simulink model "KD_cl_harness_cl_ouports_added"  (R2015b)
settings: Solver=ode45  StartTime=0  StopTime=inf  FixedStep=0.01  MaxStep=0.005  RelTol=1e-5  AbsTol=1e-5
undefined symbols (not defined in the file or in its folder): A2, bin_vec, c_0, c_1000, c_1000inv, c_100inv, c_1d2p4, c_1p7, c_4400inv, c_5500inv, c_80, c_compmap, c_ctok, c_fflow_max, c_fflow_min, c_filt, c_flowdiv, c_flowmin, c_flowmult, c_inf, c_km1d2k, c_n1, c_p00001, c_p01, c_p1e9, c_p4d1p4, c_pincomp, c_rair, c_roacorr, c_rpmtoradpers, c_svrthrottle1, c_svrthrottle2, c_svrthrottlearg, c_svrthrottlebeta, c_vnliftmax, c_vnliftmin, cl_offset, clff, Coefs, const, const_exhat, const_vec, Dual_array, dual_zero, egr_ecu_ff, expcon, f_mat, gs_jul, HQP_eps, HQP_INF, HQP_saturation, IV, L2, length_L, maxL, mHQP_saturation, minL, Newton, nRed, num_constraints ... (+22)
libraries: simulink x33
(part 6 of 6)

== system KD_cl_harness_cl_ouports_added/ctrl_rb_explicit_20140220_v6_simp/ntremap/remap_wt_to_map/ThrottleModel1/AirModel_map_use/Forward_Flow/For_Iterator_Subsystem ==
  u : Inport
  sv1 : Inport  Port=2
  sv2 : Inport  Port=3
  arg : Inport  Port=4
  beta : Inport  Port=5
  Demux : Demux  Outputs=2
  Divide : Product  Inputs=*/
  For Iterator : ForIterator  ResetStates=reset  IterationLimit=SVR_EGR_exhat.num_SV
  Gain : Gain  Gain=100
      settings: AttributesFormatString=%<Gain>
  Product{,1..3} (4 alike) : Product  RndMeth=Zero
  Saturation1 : Saturate  UpperLimit=9  LowerLimit=1
      settings: AttributesFormatString=%<LowerLimit>\n%<UpperLimit>
  Selector : Selector  InputPortWidth=SVR_EGR_exhat.num_SV  IndexOptions=Index vector (port)  Indices=[1 3]  OutputSizes=1
  Selector1 : Selector  InputPortWidth=SVR_EGR_exhat.num_SV  IndexOptions=Index vector (port)  Indices=[1 3]  OutputSizes=1
  Selector2 : Selector  InputPortWidth=SVR_EGR_exhat.num_SV  IndexOptions=Index vector (port)  Indices=[1 3]  OutputSizes=1
  Sum : Sum  Inputs=|-+
  Sum1 : Sum  Inputs=+-|
  Sum2 : Sum  Inputs=-|-
  Sum3 : Sum  Inputs=++|
  Unit Delay : UnitDelay  SampleTime=-1
  exp Lookup Table : Lookup  InputValues=SVR_EGR_exhat.exp.x  Table=SVR_EGR_exhat.exp.y  LookUpMeth=Interpolation-Use End Values
      settings: AttributesFormatString=%<LookUpMeth>\n%<InputValues>
  ba : Outport  OutDataTypeStr=single
  sat_out-65 : Outport  Port=2
  wires:
  exp Lookup Table/1 -> Product3/1
  Divide/1 -> exp Lookup Table/1
  Unit Delay/1 -> Sum3/1
  sv1/1 -> Selector/1
  sv2/1 -> Selector1/1
  beta/1 -> Selector2/1
  u/1 -> Demux/1
  Selector/1 -> Sum/1
  Demux/1 -> Sum/2
  Selector1/1 -> Sum1/2
  Demux/2 -> Sum1/1
  Sum/1 -> Product/1, Product/2
  Sum1/1 -> Product1/1, Product1/2
  Product/1 -> Sum2/1
  Product1/1 -> Sum2/2
  Sum2/1 -> Divide/1
  arg/1 -> Product2/1, Product2/2
  Product2/1 -> Gain/1
  Gain/1 -> Divide/2
  Selector2/1 -> Product3/2
  Product3/1 -> Sum3/2
  Sum3/1 -> Unit Delay/1, ba/1
  [iter] -> Selector/2
  [iter] -> Selector1/2
  [iter] -> Selector2/2
  For Iterator/1 -> Saturation1/1, sat_out-65/1
  Saturation1/1 -> [iter]

== matlab function KD_cl_harness_cl_ouports_added/EGR Valve/SVR EGR/EGR_model/Air Model_map_use/Forward-Flow/SVR_EGR ==
  data: u input; B_A_spd output; num_SV input; Beta input; SV input; arg input
function B_A_spd = fcn(u, num_SV, Beta, SV, arg)
%#eml
Kern=zeros(length(SV),1);
    for n=1:num_SV
        v = SV(n,:).';
        Kern(n)=exp(-(u-v)'*(u-v)/(50*(2*arg^2)));
    end
B_A_spd = Beta.'*Kern;

== matlab function KD_cl_harness_cl_ouports_added/Turbine/TurbineMap/TurbineMAP1 ==
  data: turb_pres_ratio input; omega_turbo input; p_in_turb input; T_ambient input; T_exh_man input; VNlift input; W_turbine_sim output; Turb_Constants input; TurbFlowCoefs input; TurbTempCoefs input; T_out_turbine output; eta_turb output; A_turbine output; phi output; delta_T_Turbo output; Tq_turbine output
 function [W_turbine_sim, T_out_turbine,eta_turb,A_turbine,phi,delta_T_Turbo,Tq_turbine] = TurbineMap(turb_pres_ratio,omega_turbo,p_in_turb,T_ambient,T_exh_man,VNlift,Turb_Constants, TurbFlowCoefs, TurbTempCoefs)

%% Reference: Turbocharger modelling for Automotive Control Applications by Paul Moraal and Ilya Kolmanovsky
% if T_exh_man <= 0
%     a = 1;
% end
Dia_turb = Turb_Constants(1); %Turbine diameter
Cp = Turb_Constants(2);  % Cp_Air_300K_KJ_per_kg_K
gamma_air = Turb_Constants(3);
eng_Vol = Turb_Constants(4);

PR= turb_pres_ratio;

%% putting saturartions on the blocks
PR = median([0.0001 PR 0.97]); % to avoid Zero-crossing errors

A_turbine  =   TurbFlowCoefs(1) +TurbFlowCoefs(2)*VNlift + TurbFlowCoefs(3)*omega_turbo +TurbFlowCoefs(4)*VNlift.^2 + TurbFlowCoefs(5)*omega_turbo.^2;

p_crit = ((gamma_air + 1)/2)^(gamma_air/(1 -gamma_air));

if PR > p_crit 
    phi_by_At = sqrt(((2*gamma_air)/(gamma_air-1))*(PR^(2/gamma_air) - PR^((gamma_air+1)/gamma_air)));
else
    phi_by_At = 0.6847;  %% check this value
end

phi = phi_by_At * A_turbine ;
phi = median([0.00001 phi 0.2]);
%%
%% to eliminate Zero crossing errors of  simulink
p_in_turb =  median([50 p_in_turb 1000]);
T_exh_man =  median([100 T_exh_man 2000]);

%%
W_turbine_sim = (phi * p_in_turb)/sqrt(T_exh_man); % kgpersec

U_by_C_den = 60*sqrt(2*Cp*T_exh_man*(1- (PR)^((gamma_air-1)/gamma_air)));

U_by_C = (pi* Dia_turb* omega_turbo)/U_by_C_den ;


delta_T_Turbo =  TurbTempCoefs(1) + TurbTempCoefs(2)*U_by_C +TurbTempCoefs(3)*PR...
    + TurbTempCoefs(4)*VNlift +TurbTempCoefs(5)*U_by_C^2 +  TurbTempCoefs(6)*PR^2 +TurbTempCoefs(7)*VNlift^2  ;

% delta_T_Turbo = median([ 0 delta_T_Turbo  250]);
T_out_turbine = T_exh_man - delta_T_Turbo;

eta_turb_num  = 1- (T_out_turbine/T_exh_man);
eta_turb_den = 1 - PR^(0.2857);
eta_turb = eta_turb_num/eta_turb_den ;

% Tq_in Newton meter
% %  Tq in N_m
Tq_turbine = (Cp*W_turbine_sim*delta_T_Turbo*60)/(2*pi*omega_turbo);

== matlab function KD_cl_harness_cl_ouports_added/Intercooler/Intercooler/MATLAB Function ==
  data: T_in_IC input; T_ambient input; T_out_IC output; ICTempCoefs input
function T_out_IC = InterCoolerMap(T_in_IC,T_ambient,ICTempCoefs)
%#codegen

delT = T_in_IC - T_ambient;
T_out_IC= ICTempCoefs(1)*delT ^2+ ICTempCoefs(2)*delT + ICTempCoefs(3);

== matlab function KD_cl_harness_cl_ouports_added/Compressor/Comp Map/MATLAB Function ==
  data: pres_Rat input; W_comp output; T_in_comp input; omega_turbo_RPM input; Comp_Constants input; CompPresRatCoefs input; CompEffCoefs input; T_out_comp output; P_comp_W output; pres_Rat1 output; Uc output; Mach output; psi output; k1 output; k2 output; k3 output; PhiC output; Comp_Efficiency output; PhiC1 output; a1 output; a2 output; a3 output; Tq_Compressor output
function [W_comp, T_out_comp,P_comp_W, pres_Rat1,Uc,Mach,psi,k1,k2,k3,PhiC,Comp_Efficiency,PhiC1,a1,a2,a3,Tq_Compressor]   = CompMap(pres_Rat,T_in_comp,omega_turbo_RPM,Comp_Constants,CompPresRatCoefs,CompEffCoefs)

%% Reference: Turbocharger modelling for Automotive Control Applications by Paul Moraal and Ilya Kolmanovsky

dc = Comp_Constants(1); % Compressor Diameter(Outer impeller diameter)
gamma_air = Comp_Constants(2);
R_air = Comp_Constants(3);   % R_specific_air_J_per_kg_kelvin
Cp_Air = Comp_Constants(4);  % Cp_Air_300K_J_per_kg_K
Rho_Air = Comp_Constants(5); % rho_Air_300K_kg_per_m3

x_low = CompPresRatCoefs(1:6);
x_high = CompPresRatCoefs(7:12);

Ntc_cutoff = 25000;
ratio = 0.5*(1 + tanh(((omega_turbo_RPM-Ntc_cutoff)*2*pi)/Ntc_cutoff));
PRcoeffs = (1-ratio)*x_low + ratio*x_high;

% pres_Rat = p_out_comp/p_in_comp;

pres_Rat1 = pres_Rat;
% pres_Rat = median([1 pres_Rat 3]);
% limit pressure ratio accordingly

%% Uc  = Blade speed
Uc = (pi/60)*dc*omega_turbo_RPM;  %% Equation 24

%% Mach = Mach Number
Mach = Uc/(sqrt(gamma_air*R_air*T_in_comp));  %% Equation 26

%% psi = slip factor
psi_num = Cp_Air*T_in_comp*((pres_Rat^((gamma_air -1)/gamma_air))-1);
psi_den = 0.5*Uc*Uc;
psi = psi_num/psi_den;   %% head parameter Equation 23
psi = median([0.0003 psi 10]);

k1 = PRcoeffs(1) + PRcoeffs(2)*Mach;
k2 = PRcoeffs(3) + PRcoeffs(4)*Mach;
k3 = PRcoeffs(5) + PRcoeffs(6)*Mach;

PhiC = ((k3*psi)-k1)/(k2+psi); %%Normalized compressor flow %% Equation 29
PhiC1 = PhiC;
W_comp = PhiC*Rho_Air*(pi/4)*dc*dc*Uc;
W_comp = median([0.0010 W_comp 0.3]);

% % Efficency Calculations

a1 = (CompEffCoefs(1) +  CompEffCoefs(2)*Mach)/(CompEffCoefs(3) - Mach);
a2 = (CompEffCoefs(4) +  CompEffCoefs(5)*Mach)/(CompEffCoefs(6) - Mach);
a3 = (CompEffCoefs(7) +  CompEffCoefs(8)*Mach)/(CompEffCoefs(9) - Mach);

% A = [a1 a2 a3];
Comp_Efficiency = a1*PhiC^2 + a2*PhiC + a3; %%Equation 27
% Comp_Efficiency = median([0.01 Comp_Efficiency 1]);


delta_T_comp = (T_in_comp/Comp_Efficiency)*(pres_Rat^((gamma_air -1)/gamma_air) - 1);
delta_T_comp = median([7  delta_T_comp 150]);

T_out_comp = T_in_comp + delta_T_comp ;  %%Equation 5

P_comp_W = W_comp*Cp_Air*delta_T_comp ; %% power in KW

%% Tq in N-m
Tq_Compressor = (Cp_Air*W_comp*delta_T_comp*60)/(2*pi*omega_turbo_RPM) ;

== matlab function KD_cl_harness_cl_ouports_added/EGR cooler/EGR Cooler/MATLAB Function ==
  data: T_in_EGR_cooler input; T_out_EGR_cooler output; T_coolant input; W_egr_valve input; EGRbypassflag input; engine_speed_RPM input; EGRCoolerTempCoefs input; EGRCoolerbypassTempCoefs input
function T_out_EGR_cooler   = EGRCoolerMap(T_in_EGR_cooler,T_coolant,W_egr_valve,EGRbypassflag,engine_speed_RPM, EGRCoolerTempCoefs,EGRCoolerbypassTempCoefs )
%#codegen

if EGRbypassflag > 1.5
    
    CoolerPercentEff =  EGRCoolerTempCoefs(1) + EGRCoolerTempCoefs(2)*T_in_EGR_cooler +EGRCoolerTempCoefs(3)*W_egr_valve  +EGRCoolerTempCoefs(4)*engine_speed_RPM...
                    +EGRCoolerTempCoefs(5)*T_in_EGR_cooler^2 + EGRCoolerTempCoefs(6)*W_egr_valve^2 + EGRCoolerTempCoefs(7)*engine_speed_RPM^2;
    
    T_out_EGR_cooler = T_in_EGR_cooler + (T_coolant - T_in_EGR_cooler)*CoolerPercentEff/100;
    
else
    T_out_EGR_cooler = EGRCoolerbypassTempCoefs(1) + EGRCoolerbypassTempCoefs(2)*T_in_EGR_cooler;

end

== matlab function KD_cl_harness_cl_ouports_added/EGR Throttle/EGR Throttle/Throttle Model2/Air Model_map_use/Back-Flow/SVR_throttle ==
  data: u input; B_A_spd output; num_SV input; Beta input; SV input; arg input
function B_A_spd = fcn(u, num_SV, Beta, SV, arg)
%#eml
Kern=zeros(length(SV),1);
    for n=1:num_SV
        v = SV(n,:).';
        Kern(n)=exp(-(u-v)'*(u-v)/(50*(2*arg^2)));
    end
B_A_spd = Beta.'*Kern;

== matlab function KD_cl_harness_cl_ouports_added/EGR Valve/SVR EGR/EGR_model/Air Model_map_use/Back-Flow/SVR_EGR ==
  data: u input; B_A_spd output; num_SV input; Beta input; SV input; arg input
function B_A_spd = fcn(u, num_SV, Beta, SV, arg)
%#eml
Kern=zeros(length(SV),1);
    for n=1:num_SV
        v = SV(n,:).';
        Kern(n)=exp(-(u-v)'*(u-v)/(50*(2*arg^2)));
    end
B_A_spd = Beta.'*Kern;

== matlab function KD_cl_harness_cl_ouports_added/EGR Throttle/EGR Throttle/Throttle Model2/Air Model_map_use/Forward-Flow/SVR_throttle ==
  data: u input; B_A_spd output; num_SV input; Beta input; SV input; arg input
function B_A_spd = fcn(u, num_SV, Beta, SV, arg)
%#eml
Kern=zeros(length(SV),1);
    for n=1:num_SV
        v = SV(n,:).';
        Kern(n)=exp(-(u-v)'*(u-v)/(50*(2*arg^2)));
    end
B_A_spd = Beta.'*Kern;

== matlab function KD_cl_harness_cl_ouports_added/Combsution/cylinder comp/MATLAB Function ==
  data: W_cyl_out output; omega_engine input; p_in_man input; p_exh_man input; T_in_man input; T_exh_man input; CylConstants input; cylFlowCoefs input; nVol output
function [W_cyl_out,nVol ]= CylinderMap(omega_engine, p_in_man,p_exh_man, T_in_man, T_exh_man,CylConstants,cylFlowCoefs)
%#codegen
% p_in_man
%% check this

%%constraints

T_exh_man =  median([100 T_exh_man 2000]);

cfs = cylFlowCoefs;
nVol = cfs(1) + cfs(2)*omega_engine + cfs(3)*omega_engine^2  + cfs(4)*p_exh_man + cfs(5)*p_in_man + cfs(6)*p_exh_man/sqrt(T_exh_man);   

W_cyl_out = (nVol * p_in_man *omega_engine *CylConstants(1))/(120*CylConstants(2) *T_in_man);

== matlab function KD_cl_harness_cl_ouports_added/Combsution/Exhaust /MATLAB Function1 ==
  data: omega_engine_rpm input; T_exhaust output; T_in_man input; W_cyl input; u_fuel input; F1_in input; ExhaustTempCoefs input
function T_exhaust    = ExhaustTemp(omega_engine_rpm, T_in_man, W_cyl ,u_fuel, F1_in, ExhaustTempCoefs)
%#codegen

% based on previous engine model fit
% %  no data for doing estimation.
fuelFrac = u_fuel/(W_cyl + u_fuel);
T_exhaust = T_in_man + (ExhaustTempCoefs(1)+ExhaustTempCoefs(2)*fuelFrac +ExhaustTempCoefs(3)*omega_engine_rpm*fuelFrac + ExhaustTempCoefs(4)*F1_in);
